simulink model "example_01"  (Simulink 8.2)
settings: Solver=FixedStepDiscrete  StartTime=0.0  StopTime=10.0  FixedStep=0.01  RelTol=1e-3
undefined symbols (not defined in the file or in its folder): sldvsubsys
libraries: simulink x5, sldvlib x4
settings Model: Creator=P  LastModifiedBy=P
settings DataIOCC: SignalLoggingSaveFormat=Dataset
settings OptimizationCC: ExpressionDepthLimit=128
settings DebuggingCC: FcnCallInpInsideContextMsg=EnableAllAsError  StateNameClashWarn=none
settings GRTTargetCC: CombineOutputUpdateFcns=on  GRTInterface=off
settings ConfigComp: Description=Design Verifier Custom Configuration Component  DVMaxProcessTime=3000  DVMaxTestCaseSteps=500  DVTestSuiteOptimization=CombinedObjectives (Nonlinear Extended)

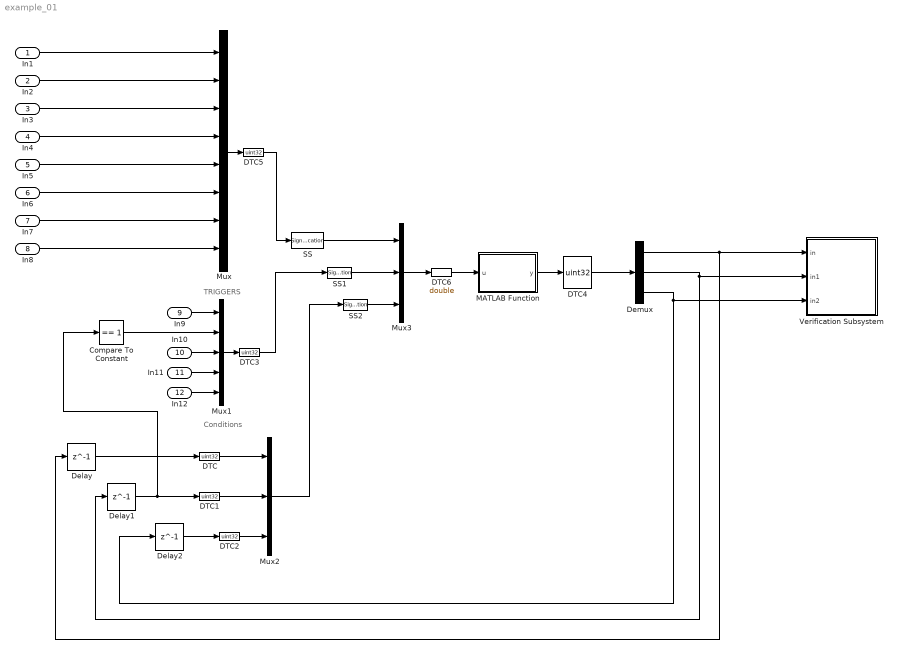
== system example_01 ==
  note: Conditions
  note: TRIGGERS
  In1 : Inport  OutDataTypeStr=boolean
  In2 : Inport  Port=2  OutDataTypeStr=boolean
  In3 : Inport  Port=3  OutDataTypeStr=boolean
  In4 : Inport  Port=4  OutDataTypeStr=boolean
  In5 : Inport  Port=5  OutDataTypeStr=boolean
  In6 : Inport  Port=6  OutDataTypeStr=boolean
  In7 : Inport  Port=7  OutDataTypeStr=boolean
  In8 : Inport  Port=8  OutDataTypeStr=boolean
  In9 : Inport  Port=9  OutDataTypeStr=boolean
  In10 : Inport  Port=10  OutDataTypeStr=boolean
  In11 : Inport  Port=11  OutDataTypeStr=boolean
  In12 : Inport  Port=12  OutDataTypeStr=boolean
  Compare To Constant : simulink/Logic and Bit Operations/Compare To Constant  relop===  const=1  OutDataTypeStr=boolean
  DTC{,1..5} (6 alike) : DataTypeConversion  OutDataTypeStr=uint32
  DTC6 : DataTypeConversion  OutDataTypeStr=double
  Delay : Delay  DelayLength=1  InitialCondition=1
  Delay1 : Delay  DelayLength=1  InitialCondition=2
  Delay2 : Delay  DelayLength=1  InitialCondition=1
  Demux : Demux  Outputs=3
  MATLAB Function : MATLAB Function  TreatAsAtomicUnit=on
  Mux : Mux  Inputs=8
  Mux1 : Mux  Inputs=5
  Mux2 : Mux  Inputs=3
  Mux3 : Mux  Inputs=3
  SS : SignalSpecification  Dimensions=8
  SS1 : SignalSpecification  Dimensions=5
  SS2 : SignalSpecification  Dimensions=3
  Verification Subsystem : Subsystem  Tag=VerificationSubsystem  DisableCoverage=on  LoadFcn=sldvsubsys('check')  TreatAsAtomicUnit=on  SimViewingDevice=on  mask(VerificationSubsystem){}
      mask init:
      | sldvsubsys('maskInit');
      settings: CopyFcn=sldvsubsys('copy');  OpenFcn=open_system(gcb,'force');
      settings: PreSaveFcn=|
      | set_param(gcb,'SimViewingDevice','on');
      | sldvsubsys('check');
      mask Help: helpview(fullfile(docroot,'toolbox','sldv','sldv.map'),'verificationsubsystem')
      mask Display: image(imread('sldvicon_versubsys.png','BackGroundColor',[1 1 1]),'center');
  wires:
  Demux/2 -> Verification Subsystem/2(in1), Delay1/1
  Delay2/1 -> DTC2/1
  Mux1/1 -> DTC3/1
  Delay1/1 -> Compare To Constant/1, DTC1/1
  Mux/1 -> DTC5/1
  Delay/1 -> DTC/1
  Mux3/1 -> DTC6/1
  Mux2/1 -> SS2/1
  Demux/1 -> Verification Subsystem/1(in), Delay/1
  In12/1 -> Mux1/5
  In7/1 -> Mux/7
  In3/1 -> Mux/3
  In2/1 -> Mux/2
  In4/1 -> Mux/4
  In5/1 -> Mux/5
  In6/1 -> Mux/6
  In8/1 -> Mux/8
  In9/1 -> Mux1/1
  In11/1 -> Mux1/4
  In10/1 -> Mux1/3
  Compare To Constant/1 -> Mux1/2
  MATLAB Function/1(y) -> DTC4/1
  Demux/3 -> Verification Subsystem/3(in2), Delay2/1
  SS/1 -> Mux3/1
  SS1/1 -> Mux3/2
  DTC4/1 -> Demux/1
  DTC/1 -> Mux2/1
  DTC1/1 -> Mux2/2
  DTC2/1 -> Mux2/3
  DTC3/1 -> SS1/1
  SS2/1 -> Mux3/3
  DTC5/1 -> SS/1
  DTC6/1 -> MATLAB Function/1(u)
  In1/1 -> Mux/1

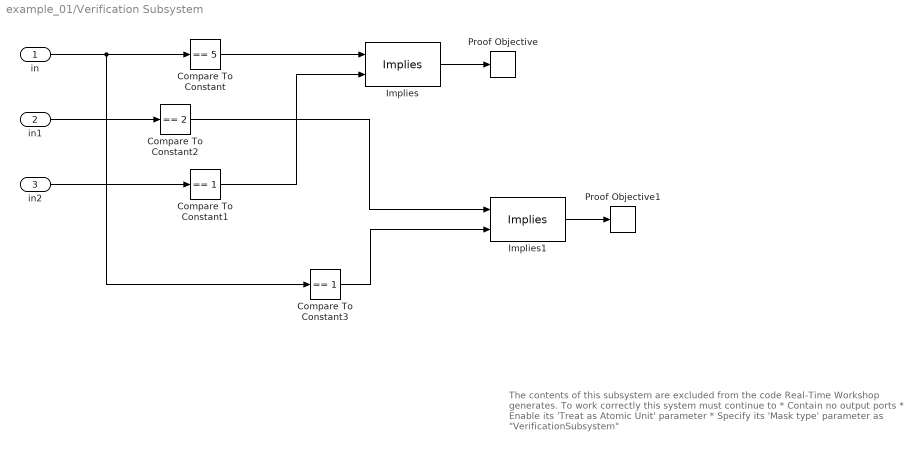
== system example_01/Verification Subsystem ==
  note: The contents of this subsystem are excluded from the code Real-Time
      | Workshop generates.
      |
      | To work correctly this system must continue to
      | * Contain no output ports
      | * Enable its 'Treat as Atomic Unit' parameter
      | * Specify its 'Mask type' parameter as "VerificationSubsystem"
  in : Inport
  in1 : Inport  Port=2
  in2 : Inport  Port=3
  Compare To Constant : simulink/Logic and Bit Operations/Compare To Constant  relop===  const=5  OutDataTypeStr=boolean
  Compare To Constant1 : simulink/Logic and Bit Operations/Compare To Constant  relop===  const=1  OutDataTypeStr=boolean
  Compare To Constant2 : simulink/Logic and Bit Operations/Compare To Constant  relop===  const=2  OutDataTypeStr=boolean
  Compare To Constant3 : simulink/Logic and Bit Operations/Compare To Constant  relop===  const=1  OutDataTypeStr=boolean
  Implies : sldvlib/Verification Utilities/Implies
  Implies1 : sldvlib/Verification Utilities/Implies
  Proof Objective : sldvlib/Objectives and Constraints/Proof Objective  enabled=on  customAVTBlockType=Proof Objective  intervals=true  dispValues=on  outEnabled=on  enableStopSim=off
      settings: AttributesFormatString=%<intervals>
  Proof Objective1 : sldvlib/Objectives and Constraints/Proof Objective  enabled=on  customAVTBlockType=Proof Objective  intervals=true  dispValues=on  outEnabled=on  enableStopSim=off
      settings: AttributesFormatString=%<intervals>
  wires:
  in/1 -> Compare To Constant3/1, Compare To Constant/1
  Compare To Constant/1 -> Implies/1
  in2/1 -> Compare To Constant1/1
  Compare To Constant1/1 -> Implies/2
  Implies/1 -> Proof Objective/1
  in1/1 -> Compare To Constant2/1
  Compare To Constant2/1 -> Implies1/1
  Compare To Constant3/1 -> Implies1/2
  Implies1/1 -> Proof Objective1/1

== matlab function MATLAB Function ==
  data: u input double; y output double
function y = fcn(u)
%#codegen
nt = 8 ; nc = 5 ;
Tr = zeros(nt,1); C = zeros(nc,1);
for i = 1:nt; Tr(i) = u(i,1); end  % Assign triggers from input U
for i = 1:nc; C(i) = u(i+nt,1); end % Assign conditions from input U
V = u(14,1);
AP = u(15,1);
AS = u(16,1);
% Assign the trigger to one based on priority
% Add additonal conditions to enable triggers here
TRIG = 0;
if  Tr(1) == 1, TRIG = 1;  % APFAIL
elseif  Tr(2) == 1, TRIG = 2;  % AP
elseif  Tr(3) == 1, TRIG = 3;  % ALTCPDN
elseif  Tr(4) == 1, TRIG = 4;  % ALTCAP
elseif  Tr(5) == 1, TRIG = 5;  % ALT
elseif  Tr(6) == 1, TRIG = 6;  % ALTS
elseif  Tr(7) == 1, TRIG = 7;  % SPD
elseif  Tr(8) == 1, TRIG = 8;  % VS
end
% 1) If in State DIS AND Trigger AP occurs THEN transit to PAH if condition C1 is True
if  (V == 1) && (TRIG == 2) && (C(1) == 1) ; V = 2;
% 2) If in State PAH AND Trigger APFAIL occurs THEN transit to DIS if condition C2 is True
elseif  (V == 2) && (TRIG == 1) && (C(2) == 1) ; V = 1;
% 3) If in State PAH AND Trigger AP occurs THEN transit to DIS if condition C2 is True
elseif  (V == 2) && (TRIG == 2) && (C(2) == 1) ; V = 1;
% 4) If in State PAH AND Trigger ALTCAP occurs THEN transit to ALTS_CAP if condition  [No Condition required] 
elseif  (V == 2) && (TRIG == 4)  ; V = 6;
% 5) If in State PAH AND Trigger ALT occurs THEN transit to ALT_HOLD if condition C5 is True
elseif  (V == 2) && (TRIG == 5) && (C(5) == 1) ; V = 5;
% 6) If in State PAH AND Trigger SPD occurs THEN transit to SPD_HOLD if condition C3 is True
elseif  (V == 2) && (TRIG == 7) && (C(3) == 1) ; V = 3;
% 7) If in State PAH AND Trigger VS occurs THEN transit to VS if condition C4 is True
elseif  (V == 2) && (TRIG == 8) && (C(4) == 1) ; V = 4;
% 8) If in State SPD_HOLD AND Trigger APFAIL occurs THEN transit to DIS if condition C2 is True
elseif  (V == 3) && (TRIG == 1) && (C(2) == 1) ; V = 1;
% 9) If in State SPD_HOLD AND Trigger AP occurs THEN transit to DIS if condition C2 is True
elseif  (V == 3) && (TRIG == 2) && (C(2) == 1) ; V = 1;
% 10) If in State SPD_HOLD AND Trigger ALTCAP occurs THEN transit to ALTS_CAP if condition  [No Condition required] 
elseif  (V == 3) && (TRIG == 4)  ; V = 6;
% 11) If in State SPD_HOLD AND Trigger ALT occurs THEN transit to ALT_HOLD if condition C5 is True
elseif  (V == 3) && (TRIG == 5) && (C(5) == 1) ; V = 5;
% 12) If in State SPD_HOLD AND Trigger SPD occurs THEN transit to PAH if condition  [No Condition required] 
elseif  (V == 3) && (TRIG == 7)  ; V = 2;
% 13) If in State SPD_HOLD AND Trigger VS occurs THEN transit to VS if condition C4 is True
elseif  (V == 3) && (TRIG == 8) && (C(4) == 1) ; V = 4;
% 14) If in State VS AND Trigger APFAIL occurs THEN transit to DIS if condition C2 is True
elseif  (V == 4) && (TRIG == 1) && (C(2) == 1) ; V = 1;
% 15) If in State VS AND Trigger AP occurs THEN transit to DIS if condition C2 is True
elseif  (V == 4) && (TRIG == 2) && (C(2) == 1) ; V = 1;
% 16) If in State VS AND Trigger ALTCAP occurs THEN transit to ALTS_CAP if condition  [No Condition required] 
elseif  (V == 4) && (TRIG == 4)  ; V = 6;
% 17) If in State VS AND Trigger ALT occurs THEN transit to ALT_HOLD if condition C5 is True
elseif  (V == 4) && (TRIG == 5) && (C(5) == 1) ; V = 5;
% 18) If in State VS AND Trigger SPD occurs THEN transit to SPD_HOLD if condition C3 is True
elseif  (V == 4) && (TRIG == 7) && (C(3) == 1) ; V = 3;
% 19) If in State VS AND Trigger VS occurs THEN transit to PAH if condition  [No Condition required] 
elseif  (V == 4) && (TRIG == 8)  ; V = 2;
% 20) If in State ALT_HOLD AND Trigger APFAIL occurs THEN transit to DIS if condition C2 is True
elseif  (V == 5) && (TRIG == 1) && (C(2) == 1) ; V = 1;
% 21) If in State ALT_HOLD AND Trigger AP occurs THEN transit to DIS if condition C2 is True
elseif  (V == 5) && (TRIG == 2) && (C(2) == 1) ; V = 1;
% 22) If in State ALT_HOLD AND Trigger ALT occurs THEN transit to PAH if condition  [No Condition required] 
elseif  (V == 5) && (TRIG == 5)  ; V = 2;
% 23) If in State ALT_HOLD AND Trigger SPD occurs THEN transit to SPD_HOLD if condition C3 is True
elseif  (V == 5) && (TRIG == 7) && (C(3) == 1) ; V = 3;
% 24) If in State ALT_HOLD AND Trigger VS occurs THEN transit to VS if condition C4 is True
elseif  (V == 5) && (TRIG == 8) && (C(4) == 1) ; V = 4;
% 25) If in State ALTS_CAP AND Trigger APFAIL occurs THEN transit to DIS if condition C2 is True
elseif  (V == 6) && (TRIG == 1) && (C(2) == 1) ; V = 1;
% 26) If in State ALTS_CAP AND Trigger AP occurs THEN transit to DIS if condition C2 is True
elseif  (V == 6) && (TRIG == 2) && (C(2) == 1) ; V = 1;
% 27) If in State ALTS_CAP AND Trigger ALTCPDN occurs THEN transit to ALT_HOLD if condition  [No Condition required] 
elseif  (V == 6) && (TRIG == 3)  ; V = 5;
% 28) If in State ALTS_CAP AND Trigger ALT occurs THEN transit to ALT_HOLD if condition C5 is True
elseif  (V == 6) && (TRIG == 5) && (C(5) == 1) ; V = 5;
end     
%   ================================================
  
% 29) If in State APON AND Trigger APFAIL occurs THEN transit to APOFF if condition  [No Condition required] 
if  (AP == 1) && (TRIG == 1)  ; AP = 2;
% 30) If in State APON AND Trigger AP occurs THEN transit to APOFF if condition  [No Condition required] 
elseif  (AP == 1) && (TRIG == 2)  ; AP = 2;
% 31) If in State APOFF AND Trigger AP occurs THEN transit to APON if condition C1 is True
elseif  (AP == 2) && (TRIG == 2) && (C(1) == 1) ; AP = 1;
end     
%   ================================================
  
% 32) If in State ALTSOFF AND Trigger ALTS occurs THEN transit to ALTSARM if condition  [No Condition required] 
if  (AS == 1) && (TRIG == 6)  ; AS = 2;
% 33) If in State ALTSARM AND Trigger APFAIL occurs THEN transit to ALTSOFF if condition C2 is True
elseif  (AS == 2) && (TRIG == 1) && (C(2) == 1) ; AS = 1;
% 34) If in State ALTSARM AND Trigger AP occurs THEN transit to ALTSOFF if condition C2 is True
elseif  (AS == 2) && (TRIG == 2) && (C(2) == 1) ; AS = 1;
% 35) If in State ALTSARM AND Trigger ALTCAP occurs THEN transit to ALTSCAP if condition  [No Condition required] 
elseif  (AS == 2) && (TRIG == 4)  ; AS = 3;
% 36) If in State ALTSARM AND Trigger ALT occurs THEN transit to ALTSOFF if condition C5 is True
elseif  (AS == 2) && (TRIG == 5) && (C(5) == 1) ; AS = 1;
% 37) If in State ALTSARM AND Trigger ALTS occurs THEN transit to ALTSOFF if condition  [No Condition required] 
elseif  (AS == 2) && (TRIG == 6)  ; AS = 1;
% 38) If in State ALTSCAP AND Trigger APFAIL occurs THEN transit to ALTSOFF if condition C2 is True
elseif  (AS == 3) && (TRIG == 1) && (C(2) == 1) ; AS = 1;
% 39) If in State ALTSCAP AND Trigger AP occurs THEN transit to ALTSOFF if condition C2 is True
elseif  (AS == 3) && (TRIG == 2) && (C(2) == 1) ; AS = 1;
% 40) If in State ALTSCAP AND Trigger ALTCPDN occurs THEN transit to ALTSOFF if condition  [No Condition required] 
elseif  (AS == 3) && (TRIG == 3)  ; AS = 1;
% 41) If in State ALTSCAP AND Trigger ALT occurs THEN transit to ALTSOFF if condition C5 is True
elseif  (AS == 3) && (TRIG == 5) && (C(5) == 1) ; AS = 1;
end     
%   ================================================
  
% ============== Set the outputs ===========
y = zeros(3,1);
y(1) = V;
y(2) = AP;
y(3) = AS;
